simulink library "util_common_lib"  (R2014b)
settings: Solver=ode45  SolverMode=SingleTasking  StartTime=0.0  StopTime=10.0  RelTol=1e-3
undefined symbols (not defined in the file or in its folder): enum_boolean, sc_msgid, sc_start_rts_id, start
undefined symbols (not defined in the file): Initial_MET, slope, util_noise_generator_sample_time
libraries: simulink x13, util_info_lib x12, util_common_lib x5
settings Model: Creator=dviazzo  LastModifiedBy=mstewart

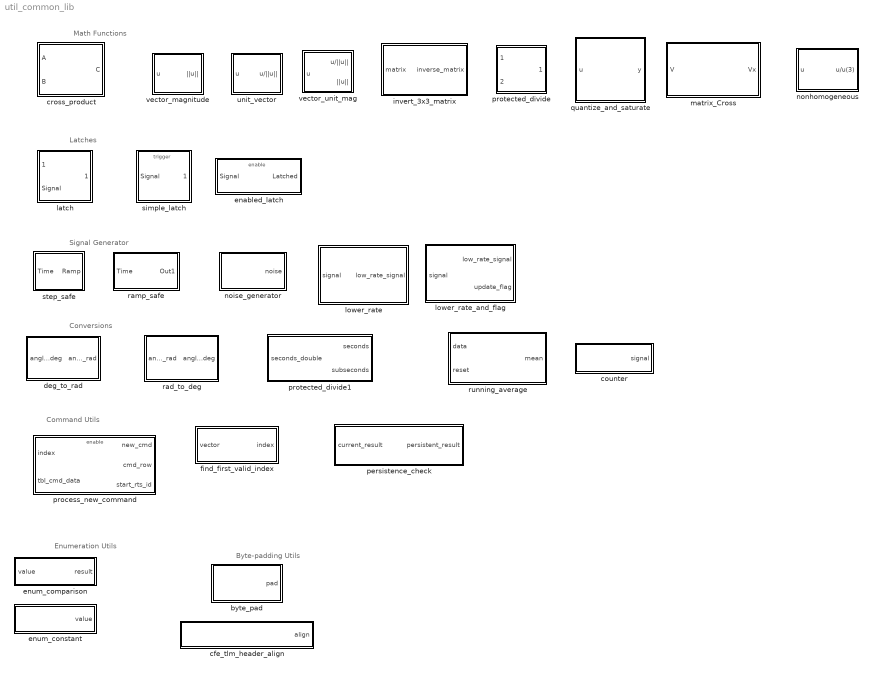
== system util_common_lib ==
  note: Enumeration Utils
  note: Command Utils
  note: Math Functions
  note: Latches
  note: Signal Generator
  note: Conversions
  note: Byte-padding Utils
  byte_pad : Subsystem  mask{n_bytes=1}
      mask prompts: n_bytes "Number of byes to pad"
      mask Display:
      | fprintf('pad %i bytes', n_bytes)
      | 
      | color('blue')
      | text(0.05,0.02,'moonex',...
      |  	'HorizontalAlignment','Left',...
      | 	'VerticalAlignment','bottom')
  cfe_tlm_header_align : Subsystem
      mask Display:
      | disp('cFE Telemetry Header Align');
      | 
      | color('blue')
      | text(0.05,0.02,'moonex',...
      |  	'HorizontalAlignment','Left',...
      | 	'VerticalAlignment','bottom')
  counter : Subsystem  TreatAsAtomicUnit=on  mask{n=0}
      mask prompts: n "Counter cycles (in ticks)"
      mask Display:
      | color('blue')
      | text(0.05,0.02,'MoonEx',...
      |  	'HorizontalAlignment','Left',...
      | 	'VerticalAlignment','bottom')
  cross_product : Subsystem
      mask Display:
      | text(.5,.5,'Cross\nProduct\nC = AxB', ...
      | 	'HorizontalAlignment','Center',...
      | 	'VerticalAlignment','middle')
      | color('blue')
      | text(0.05,0.02,'NASA',...
      |  	'HorizontalAlignment','Left',...
      | 	'VerticalAlignment','bottom')
  deg_to_rad : Subsystem
      mask Display:
      | disp('radians\ndegrees')
      | 
      | plot([.3 .7],[.47 .47])
      | 
      | color('blue')
      | text(0.05,0.02,'NASA',...
      |  	'HorizontalAlignment','Left',...
      | 	'VerticalAlignment','bottom')
  enabled_latch : Subsystem  mask{initial_output=0}
      mask prompts: initial_output "Initial Output Value"
      mask Display:
      | color('blue')
      | text(0.05,0.02,'NASA',...
      |  	'HorizontalAlignment','Left',...
      | 	'VerticalAlignment','bottom')
  enum_comparison : Subsystem  mask{comparison_type=~=, enum_type=enum_boolean, enum_value=FALSE}
      mask prompts: comparison_type "Relational Operator:"; enum_type "Enumeration Type:"; enum_value "Enumeration Value:"
      mask help:
      | Compares the incoming signal to an enumerated type.
      |
      | Once you change the enumeration type, the value selection will become disabled and you MUST close and reopen the dialog to reenable it.
      mask init:
      | rtw_data = get_param(gcb,'RTWData');  % Non-Persistent Data
      | user_data = get_param(gcb,'UserData'); % Persistent Data
      | 
      | mask_styles = get_param(gcb, 'MaskStyles');
      | 
      | if isempty(rtw_data)
      |     mask_styles{2} = user_data.type_popup;
      |     mask_styles{3} = user_data.value_popup;
      |     
      |     set_param(gcb, 'MaskStyles', mask_styles);
      |     set_param(gcb, 'enum_type', user_data.type);
      |     set_param(gcb, 'enum_value', user_data.value);
      |     
      |     if ~strcmp(gcb,'util_common_lib/enum_comparison')
      |         rtw_data.loaded = 'true';
      |     end
      |     set_param(gcb, 'RTWData', rtw_data);
      | else
      |     user_data.type_popup = mask_styles{2};
      |     user_data.value_popup = mask_styles{3};
      |     user_data.type = enum_type;
      |     user_data.value = enum_value;
      |     set_param(gcb, 'UserData', user_data);
      | end
      | 
      | mask_enables = get_param(gcb, 'MaskEnables');
      | 
      | % Make sure the user isn't selecting '...' on purpose.
      | if strcmp(enum_value, '...')
      |     if ~strcmp(mask_enables{3}, 'off')
      |         error('You must select a value.');
      |     end
      | else
      |     % Figure out the native type we're casting to
      |     enum_parents = superclasses(enum_type);
      |     bus_type = enum_parents{1};
      | 
      |     % Build up the constant string and update the inner compare block
      |     const_string = [ bus_type '(' enum_type '.' lower(enum_value) ')' ];
      |     set_param([gcb '/comparison'], 'const', const_string);
      |     set_param([gcb '/comparison'], 'relop', comparison_type);
      | end
      | 
      | clear rtw_data user_data mask_styles mask_enables enum_parents bus_type const_string
      mask TypeOptions comparison_type: == | ~=
      mask TypeOptions enum_type: enum_ap_state | enum_boolean | enum_burn_type | enum_mode | enum_reference_frame | enum_submode | enum_thruster_type
      mask Callback enum_type:
      | % Generate a list of enumeration files
      | nimbus_root = getenv('NIMBUS_ROOT');
      | enum_files = dir(fullfile(nimbus_root,'fsw','cmp','enums','*.m'));
      | % Extract the enum names into a cell array
      | enum_types = strrep({enum_files.name},'.m','');
      | 
      | user_data = get_param(gcb,'UserData');
      | 
      | % Build the popup of enum types
      | user_data.type_popup = ['popup(' strjoin(enum_types ,'|') ')'];
      | 
      | % Get current mask values
      | mask_values = get_param(gcb, 'MaskValues');
      | % Get a list of values the currently selected enumeration can take on
      | [~, enum_values] = enumeration(mask_values{2});
      | 
      | % Transpose enum_values and add in '...' so all enums share one field
      | enum_values = upper(['...' enum_values']);
      | % Construct the popup string for the enm values
      | user_data.value_popup = ['popup(' strjoin(enum_values, '|') ')'];
      | 
      | % Get the current mask styles and set the new enum type popup
      | mask_styles = get_param(gcb, 'MaskStyles');
      | mask_styles{2} = user_data.type_popup;
      | 
      | % If our determined values match the current style, the current popup
      | % is good and we can enable selection.
      | if strcmp(user_data.value_popup, mask_styles{3})
      |     set_param(gcb, 'MaskEnables', {'on';'on';'on'});
      | else
      |     % Otherwise disable the enum value popup and update its value. We have
      |     % to set the value to ... as an intermediate step to keep the window
      |     % from closing on us
      |     mask_styles{3} = user_data.value_popup;
      |     mask_values{3} = '...';
      |     set_param(gcb, 'MaskEnables', {'on';'on';'off'});
      |     set_param(gcb, 'MaskValues', mask_values);
      | end
      | 
      | % Send out the finalized mask styles
      | set_param(gcb, 'MaskStyles', mask_styles);
      | set_param(gcb, 'UserData', user_data);
      mask TypeOptions enum_value: ... | FALSE | TRUE
      mask Display: disp([comparison_type ' ' enum_value]);
  enum_constant : Subsystem  mask{enum_type=enum_boolean, enum_value=FALSE}
      mask prompts: enum_type "Enumeration Type:"; enum_value "Enumeration Value:"
      mask help:
      | Compares the incoming signal to an enumerated type.
      |
      | Once you change the enumeration type, the value selection will become disabled and you MUST close and reopen the dialog to reenable it.
      mask init:
      | rtw_data = get_param(gcb,'RTWData');  % Non-Persistent Data
      | user_data = get_param(gcb,'UserData'); % Persistent Data
      | 
      | mask_styles = get_param(gcb, 'MaskStyles');
      | 
      | if isempty(rtw_data)
      |     mask_styles{1} = user_data.type_popup;
      |     mask_styles{2} = user_data.value_popup;
      |     
      |     set_param(gcb, 'MaskStyles', mask_styles);
      |     set_param(gcb, 'enum_type', user_data.type);
      |     set_param(gcb, 'enum_value', user_data.value);
      |     
      |     if ~strcmp(gcb,'util_common_lib/enum_constant')
      |         rtw_data.loaded = 'true';
      |     end
      |     set_param(gcb, 'RTWData', rtw_data);
      | else
      |     user_data.type_popup = mask_styles{1};
      |     user_data.value_popup = mask_styles{2};
      |     user_data.type = enum_type;
      |     user_data.value = enum_value;
      |     set_param(gcb, 'UserData', user_data);
      | end
      | 
      | mask_enables = get_param(gcb, 'MaskEnables');
      | 
      | % Make sure the user isn't selecting '...' on purpose.
      | if strcmp(enum_value, '...')
      |     if ~strcmp(mask_enables{2}, 'off')
      |         error('You must select a value.');
      |     end
      | else
      |     % Figure out the native type we're casting to
      |     enum_parents = superclasses(enum_type);
      |     bus_type = enum_parents{1};
      | 
      |     % Build up the constant string and update the inner compare block
      |     const_string = [ bus_type '(' enum_type '.' lower(enum_value) ')' ];
      |     set_param([gcb '/constant'], 'Value', const_string);
      | end
      | 
      | 
      | clear rtw_data user_data mask_styles mask_enables enum_parents bus_type const_string
      mask TypeOptions enum_type: enum_ap_state | enum_boolean | enum_burn_type | enum_mode | enum_reference_frame | enum_submode | enum_thruster_type
      mask Callback enum_type:
      | % Generate a list of enumeration files
      | nimbus_root = getenv('NIMBUS_ROOT');
      | enum_files = dir(fullfile(nimbus_root,'fsw','cmp','enums','*.m'));
      | % Extract the enum names into a cell array
      | enum_types = strrep({enum_files.name},'.m','');
      | 
      | user_data = get_param(gcb,'UserData');
      | 
      | % Build the popup of enum types
      | user_data.type_popup = ['popup(' strjoin(enum_types ,'|') ')'];
      | 
      | % Get current mask values
      | mask_values = get_param(gcb, 'MaskValues');
      | % Get a list of values the currently selected enumeration can take on
      | [~, enum_values] = enumeration(mask_values{1});
      | 
      | % Transpose enum_values and add in '...' so all enums share one field
      | enum_values = upper(['...' enum_values']);
      | % Construct the popup string for the enm values
      | user_data.value_popup = ['popup(' strjoin(enum_values, '|') ')'];
      | 
      | % Get the current mask styles and set the new enum type popup
      | mask_styles = get_param(gcb, 'MaskStyles');
      | mask_styles{1} = user_data.type_popup;
      | 
      | % If our determined values match the current style, the current popup
      | % is good and we can enable selection.
      | if strcmp(user_data.value_popup, mask_styles{2})
      |     set_param(gcb, 'MaskEnables', {'on';'on'});
      | else
      |     % Otherwise disable the enum value popup and update its value. We have
      |     % to set the value to ... as an intermediate step to keep the window
      |     % from closing on us
      |     mask_styles{2} = user_data.value_popup;
      |     mask_values{2} = '...';
      |     set_param(gcb, 'MaskEnables', {'on';'off'});
      |     set_param(gcb, 'MaskValues', mask_values);
      | end
      | 
      | % Send out the finalized mask styles
      | set_param(gcb, 'MaskStyles', mask_styles);
      | set_param(gcb, 'UserData', user_data);
      mask TypeOptions enum_value: ... | FALSE | TRUE
      mask Display: disp(enum_value);
  find_first_valid_index : Subsystem  mask{vector_length=2}
      mask prompts: vector_length "Length of vector input"
      mask Display:
      | color('blue')
      | text(0.05,0.02,'MoonEx',...
      |  	'HorizontalAlignment','Left',...
      | 	'VerticalAlignment','bottom')
  invert_3x3_matrix : Subsystem
      mask Display:
      | disp('Inverse(A)\n(3x3)')
      | 
      | color('blue')
      | text(0.05,0.02,'NASA',...
      |  	'HorizontalAlignment','Left',...
      | 	'VerticalAlignment','bottom')
  latch : Subsystem  mask{Initial_Latch=[0 Initial_MET]}
      mask prompts: Initial_Latch "Initial Output Value"
      mask init:
      | if isempty(Initial_Latch)
      |    Initial_Latch = 0;
      | end
      mask Display:
      | color('blue')
      | text(0.05,0.02,'NASA',...
      |  	'HorizontalAlignment','Left',...
      | 	'VerticalAlignment','bottom')
  lower_rate : Subsystem  mask{counter_max=10, counter_init=0}
      mask prompts: counter_max "Counter maximum value (model freq / block freq)"; counter_init "Counter Initial Value"
      mask Display:
      | color('blue')
      | text(0.05,0.02,'MoonEx',...
      |  	'HorizontalAlignment','Left',...
      | 	'VerticalAlignment','bottom')
  lower_rate_and_flag : Subsystem  mask{counter_max=1, counter_init=[]}
      mask prompts: counter_max "Counter maximum value (model freq / block freq)"; counter_init "Counter initial value"
      mask Display:
      | color('blue')
      | text(0.05,0.02,'MoonEx',...
      |  	'HorizontalAlignment','Left',...
      | 	'VerticalAlignment','bottom')
  matrix_Cross : Subsystem
      mask Display:
      | text(.5,.5,'Cross\nMatrix\nV -> Vx', ...
      | 	'HorizontalAlignment','Center',...
      | 	'VerticalAlignment','middle')
      | color('blue')
      | text(0.05,0.02,'NASA',...
      |  	'HorizontalAlignment','Left',...
      | 	'VerticalAlignment','bottom')
  noise_generator : Subsystem  mask(noise_generator){std_dev=, bias=, seed=, on=1, sample_time=util_noise_generator_sample_time}
      mask prompts: std_dev "std deviation"; sample_time "sample time"
      mask help: Outputs a noise signal.
      mask init:
      | null_vector=zeros(size(std_dev));
      mask Display:
      | color('blue')
      | text(0.05,0.02,'NASA',...
      |  	'HorizontalAlignment','Left',...
      | 	'VerticalAlignment','bottom')
  nonhomogeneous : Subsystem
      mask Display:
      | color('blue')
      | text(0.05,0.02,'NASA',...
      |  	'HorizontalAlignment','Left',...
      | 	'VerticalAlignment','bottom')
  persistence_check : Subsystem  mask{persistence_limit=10}
      mask prompts: persistence_limit "Persistence Limit (counter initialize at zero)"
      mask Display:
      | color('blue')
      | text(0.05,0.02,'MoonEx',...
      |  	'HorizontalAlignment','Left',...
      | 	'VerticalAlignment','bottom')
  process_new_command : Subsystem  TreatAsAtomicUnit=on
      mask Display:
      | color('blue')
      | text(0.05,0.02,'MoonEx',...
      |  	'HorizontalAlignment','Left',...
      | 	'VerticalAlignment','bottom')
  protected_divide : Subsystem  mask{fault_value=0, tolerance=eps}
      mask prompts: fault_value "Fault value to be output when div by zero occurs"; tolerance "Tolerance for divisor below which fault is declared"
      mask Display:
      | color('blue')
      | text(0.05,0.02,'MoonEx',...
      |  	'HorizontalAlignment','Left',...
      | 	'VerticalAlignment','bottom')
      | 
      | color('black')
      | port_label('input', 1, '*')
      | port_label('input', 2, '/')
      | 
      | port_label('output', 1, '>')
      | 
      | disp('divide')
  protected_divide1 : Subsystem
      mask Display:
      | color('blue')
      | text(0.05,0.02,'MoonEx',...
      |  	'HorizontalAlignment','Left',...
      | 	'VerticalAlignment','bottom')
      | 
      | color('black')
      | port_label('input', 1, 't')
      | 
      | port_label('output', 1, 'secs')
      | port_label('output', 2, 'subs')
      | 
      | disp('6byte time')
  quantize_and_saturate : Subsystem  mask(PWL-Palette){RES=1, OPER=truncate, out_min=-inf, out_max=inf}
      mask prompts: RES "Resolution:"; OPER "Type"; out_min "Output Minimum"; out_max "Output Maximum"
      mask init:
      | x=[-5:.1:5];operator={'round';'fix';'floor';'ceil'};
      | y=feval(operator{OPER},x);
      | if(isfinite(out_max))
      |    y(find(y>3))=3;
      | end
      | if(isfinite(out_min))
      |    y(find(y<-3))=-3;
      | end
      | [xx,yy]=stairs(x,y);
      | set_param([gcb '/Type'],'Operator',operator{OPER});
      mask TypeOptions OPER: round | truncate | floor | ceil
      mask Display:
      | plot([0 0],[-4,4],[-4,4],[0 0],xx,yy)
      | color('blue')
      | text(1.5,-5,'NASA',...
      |  	'HorizontalAlignment','Left',...
      | 	'VerticalAlignment','bottom')
  rad_to_deg : Subsystem
      mask Display:
      | disp('degrees\nradians')
      | 
      | plot([.3 .7],[.47 .47])
      | 
      | color('blue')
      | text(0.05,0.02,'NASA',...
      |  	'HorizontalAlignment','Left',...
      | 	'VerticalAlignment','bottom')
  ramp_safe : Subsystem  mask(Ramp){slope=, start=, X0=, VectorParams1D=on}
      mask prompts: start "Start time:"; X0 "Initial output:"; VectorParams1D "Interpret vector parameters as 1-D"
      mask help: Output a ramp signal starting at the specified time.
      mask Display:
      | plot([0:10],[.001,.001,.001,.001,.001,1:6])
      | 
      | color('blue')
      | text(0.05,0.02,'NASA',...
      |  	'HorizontalAlignment','Left',...
      | 	'VerticalAlignment','bottom')
  running_average : Subsystem  mask{initial_mean=[0 0 0]}
      mask prompts: initial_mean "initial mean value:"
      mask Display:
      | color('blue')
      | text(0.05,0.02,'MoonEx',...
      |  	'HorizontalAlignment','Left',...
      | 	'VerticalAlignment','bottom')
  simple_latch : Subsystem
      mask Display:
      | color('blue')
      | text(0.05,0.02,'NASA',...
      |  	'HorizontalAlignment','Left',...
      | 	'VerticalAlignment','bottom')
  step_safe : Subsystem  mask{step_time=start, initial_value=0, final_value=slope}
      mask prompts: step_time "Step time:"; initial_value "Initial value:"; final_value "Final value:"
      mask Display:
      | plot([0,.5,.5,1],[.001,.001,.999,.999])
      | 
      | color('blue')
      | text(0.05,0.02,'NASA',...
      |  	'HorizontalAlignment','Left',...
      | 	'VerticalAlignment','bottom')
  unit_vector : Subsystem
      mask Display:
      | color('blue')
      | text(0.05,0.02,'NASA',...
      |  	'HorizontalAlignment','Left',...
      | 	'VerticalAlignment','bottom')
  vector_magnitude : Subsystem
      mask Display:
      | port_label('input',1,'u')
      | port_label('output',1,'||u||')
      | color('blue')
      | text(0.05,0.02,'NASA',...
      |  	'HorizontalAlignment','Left',...
      | 	'VerticalAlignment','bottom')
  vector_unit_mag : Subsystem
      mask Display:
      | color('blue')
      | text(0.05,0.02,'NASA',...
      |  	'HorizontalAlignment','Left',...
      | 	'VerticalAlignment','bottom')

== system util_common_lib/byte_pad ==
  note: Extremely explicit signal typing for uint8s of variable size for message padding
  Constant : Constant  Value=zeros(1,n_bytes)  OutDataTypeStr=uint8
  Data Type Conversion : DataTypeConversion  OutDataTypeStr=uint8
  Library Information : util_info_lib/Library Information  owner='NONE'
  pad : Outport
  wires:
  Constant/1 -> Data Type Conversion/1
  Data Type Conversion/1 -> pad/1

== system util_common_lib/cfe_tlm_header_align ==
  Constant : Constant  Value=zeros(1,4)  OutDataTypeStr=uint8
  Data Type Conversion : DataTypeConversion  OutDataTypeStr=uint8
  Library Information : util_info_lib/Library Information  owner='NONE'
  align : Outport
  wires:
  Data Type Conversion/1 -> align/1
  Constant/1 -> Data Type Conversion/1

== system util_common_lib/counter ==
  Bias : Bias  Bias=1
  Compare To Constant : simulink/Logic and Bit Operations/Compare To Constant  relop=>=  const=n  OutDataTypeStr=uint8
  Library Information : util_info_lib/Library Information  owner='NONE'
  Memory : Memory  X0=n  InheritSampleTime=on
  Switch6 : Switch  Criteria=u2 ~= 0  InputSameDT=on
  constant1 : Constant  Value=0
  signal : Outport
  wires:
  constant1/1 -> Switch6/1
  Bias/1 -> Compare To Constant/1, Switch6/3
  Compare To Constant/1 -> Switch6/2, signal/1
  Switch6/1 -> Memory/1
  Memory/1 -> Bias/1

== system util_common_lib/cross_product ==
  A : Inport
  B : Inport  Port=2
  Vector Concatenate : Concatenate  NumInputs=3
  Vector Concatenate1 : Concatenate
  i axis : Fcn  Expr=u(2)*u(6)-u(5)*u(3)
  j axis : Fcn  Expr=u(4)*u(3)-u(1)*u(6)
  k axis : Fcn  Expr=u(1)*u(5)-u(4)*u(2)
  C : Outport
  wires:
  B/1 -> Vector Concatenate1/2
  Vector Concatenate/1 -> C/1
  A/1 -> Vector Concatenate1/1
  k axis/1 -> Vector Concatenate/3
  j axis/1 -> Vector Concatenate/2
  i axis/1 -> Vector Concatenate/1
  Vector Concatenate1/1 -> k axis/1, j axis/1, i axis/1

== system util_common_lib/deg_to_rad ==
  angle_in_deg : Inport
  Gain : Gain  Gain=0.017453292519943295474371680598
  angle_in_rad : Outport
  wires:
  angle_in_deg/1 -> Gain/1
  Gain/1 -> angle_in_rad/1

== system util_common_lib/enabled_latch ==
  Signal : Inport
  Enable : EnablePort
  Latched : Outport  InitialOutput=initial_output
  wires:
  Signal/1 -> Latched/1

== system util_common_lib/enum_comparison ==
  value : Inport
  Library Information : util_info_lib/Library Information  owner='NONE'
  comparison : simulink/Logic and Bit Operations/Compare To Constant  relop=~=  const=uint8(enum_boolean.false)  OutDataTypeStr=boolean
  result : Outport
  wires:
  value/1 -> comparison/1
  comparison/1 -> result/1

== system util_common_lib/enum_constant ==
  Library Information : util_info_lib/Library Information  owner='NONE'
  constant : Constant  Value=uint8(enum_boolean.false)
  value : Outport
  wires:
  constant/1 -> value/1

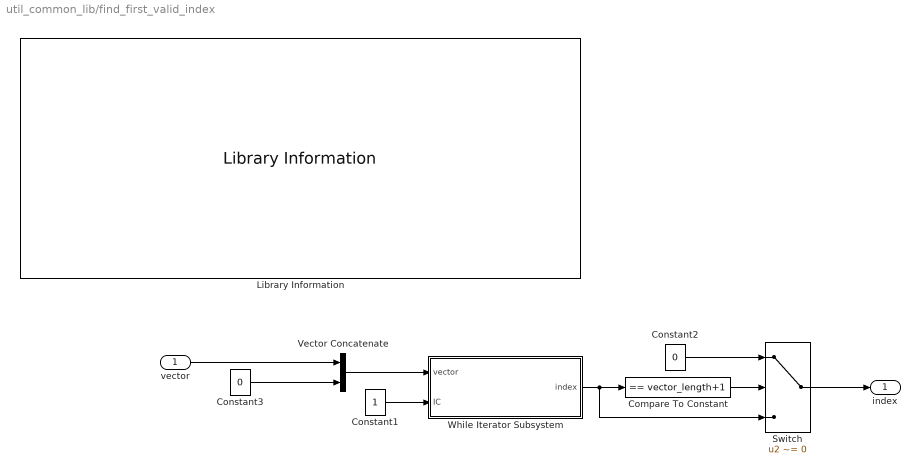
== system util_common_lib/find_first_valid_index ==
  vector : Inport
  Compare To Constant : simulink/Logic and Bit Operations/Compare To Constant  relop===  const=vector_length+1  OutDataTypeStr=boolean
  Constant1 : Constant  OutDataTypeStr=uint8
  Constant2 : Constant  Value=0  OutDataTypeStr=uint32
  Constant3 : Constant  Value=0  OutDataTypeStr=Inherit: Inherit via back propagation
  Library Information : util_info_lib/Library Information  owner='NONE'
  Switch : Switch  Criteria=u2 ~= 0
  Vector Concatenate : Concatenate
  While Iterator Subsystem : Subsystem  TreatAsAtomicUnit=on
  index : Outport
  wires:
  Constant3/1 -> Vector Concatenate/2
  Vector Concatenate/1 -> While Iterator Subsystem/1(vector)
  vector/1 -> Vector Concatenate/1
  Switch/1 -> index/1
  Constant2/1 -> Switch/1
  Compare To Constant/1 -> Switch/2
  While Iterator Subsystem/1(index) -> Compare To Constant/1, Switch/3
  Constant1/1 -> While Iterator Subsystem/2(IC)

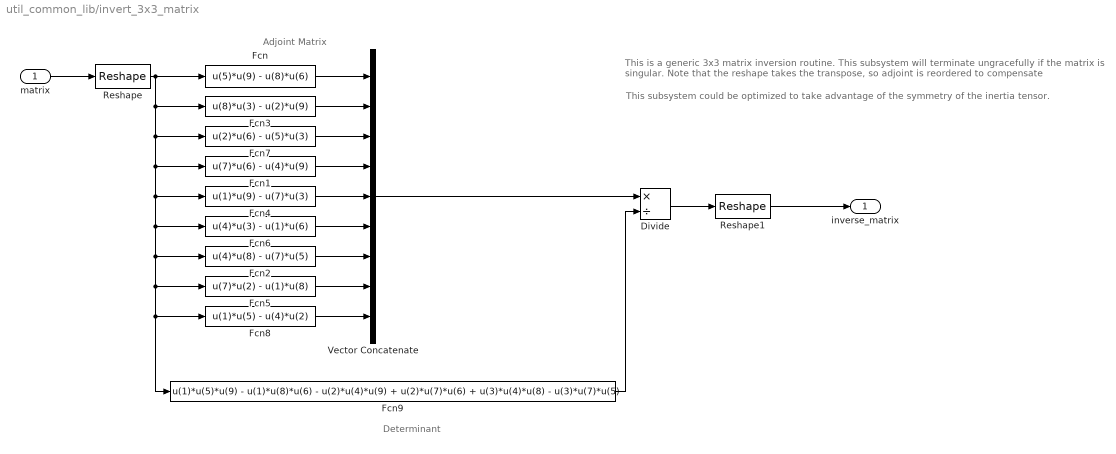
== system util_common_lib/invert_3x3_matrix ==
  note: Adjoint Matrix
  note: Determinant
  note: This is a generic 3x3 matrix inversion routine.
      | This subsystem will terminate ungracefully if the matrix is singular.
      | Note that the reshape takes the transpose, so adjoint is reordered to compensate
  note: This subsystem could be optimized to take advantage of the symmetry of the inertia tensor.
  matrix : Inport
  Divide : Product  Inputs=*/
  Fcn : Fcn  Expr=u(5)*u(9) - u(8)*u(6)
  Fcn1 : Fcn  Expr=u(7)*u(6) - u(4)*u(9)
  Fcn2 : Fcn  Expr=u(4)*u(8) - u(7)*u(5)
  Fcn3 : Fcn  Expr=u(8)*u(3) - u(2)*u(9)
  Fcn4 : Fcn  Expr=u(1)*u(9) - u(7)*u(3)
  Fcn5 : Fcn  Expr=u(7)*u(2) - u(1)*u(8)
  Fcn6 : Fcn  Expr=u(4)*u(3) - u(1)*u(6)
  Fcn7 : Fcn  Expr=u(2)*u(6) - u(5)*u(3)
  Fcn8 : Fcn  Expr=u(1)*u(5) - u(4)*u(2)
  Fcn9 : Fcn  Expr=u(1)*u(5)*u(9) - u(1)*u(8)*u(6) - u(2)*u(4)*u(9) + u(2)*u(7)*u(6) + u(3)*u(4)*u(8) - u(3)*u(7)*u(5)
  Reshape : Reshape  OutputDimensionality=Row vector (2-D)
  Reshape1 : Reshape  OutputDimensionality=Customize  OutputDimensions=[3,3]
  Vector Concatenate : Concatenate  NumInputs=9
  inverse_matrix : Outport
  wires:
  matrix/1 -> Reshape/1
  Fcn9/1 -> Divide/2
  Reshape/1 -> Fcn/1, Fcn3/1, Fcn7/1, Fcn1/1, Fcn4/1, Fcn6/1, Fcn2/1, Fcn5/1, Fcn9/1, Fcn8/1
  Divide/1 -> Reshape1/1
  Reshape1/1 -> inverse_matrix/1
  Fcn/1 -> Vector Concatenate/1
  Fcn3/1 -> Vector Concatenate/2
  Fcn7/1 -> Vector Concatenate/3
  Fcn1/1 -> Vector Concatenate/4
  Fcn4/1 -> Vector Concatenate/5
  Fcn6/1 -> Vector Concatenate/6
  Fcn2/1 -> Vector Concatenate/7
  Fcn5/1 -> Vector Concatenate/8
  Fcn8/1 -> Vector Concatenate/9
  Vector Concatenate/1 -> Divide/1

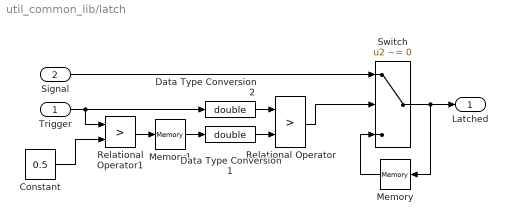
== system util_common_lib/latch ==
  Trigger : Inport
  Signal : Inport  Port=2
  Constant : Constant  Value=0.5
  Data Type Conversion1 : DataTypeConversion  OutDataTypeStr=double
  Data Type Conversion2 : DataTypeConversion  OutDataTypeStr=double
  Memory : Memory  X0=Initial_Latch  InheritSampleTime=on
  Memory1 : Memory  InheritSampleTime=on
  Relational Operator : RelationalOperator  Operator=>  OutDataTypeStr=boolean
  Relational Operator1 : RelationalOperator  Operator=>  OutDataTypeStr=boolean
  Switch : Switch  Criteria=u2 ~= 0  InputSameDT=on
  Latched : Outport
  wires:
  Trigger/1 -> Data Type Conversion2/1, Relational Operator1/1
  Relational Operator1/1 -> Memory1/1
  Memory/1 -> Switch/3
  Signal/1 -> Switch/1
  Switch/1 -> Latched/1, Memory/1
  Constant/1 -> Relational Operator1/2
  Data Type Conversion2/1 -> Relational Operator/1
  Memory1/1 -> Data Type Conversion1/1
  Data Type Conversion1/1 -> Relational Operator/2
  Relational Operator/1 -> Switch/2

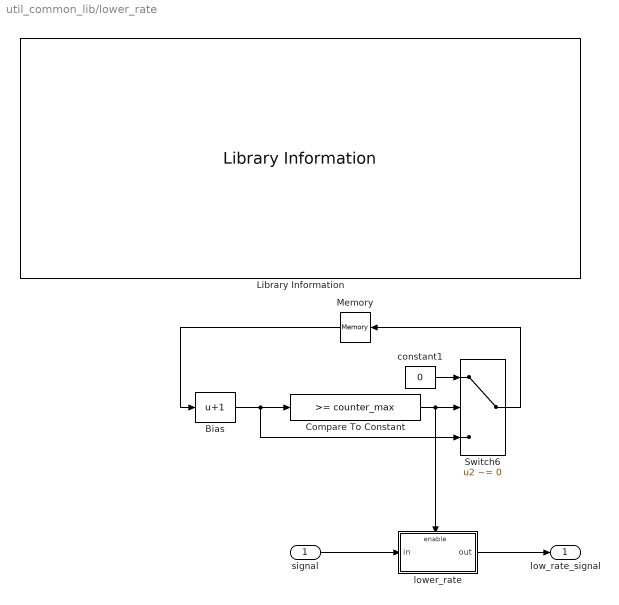
== system util_common_lib/lower_rate ==
  signal : Inport
  Bias : Bias  Bias=1
  Compare To Constant : simulink/Logic and Bit Operations/Compare To Constant  relop=>=  const=counter_max  OutDataTypeStr=uint8
  Library Information : util_info_lib/Library Information  owner='NONE'
  Memory : Memory  X0=counter_init  InheritSampleTime=on
  Switch6 : Switch  Criteria=u2 ~= 0  InputSameDT=on
  constant1 : Constant  Value=0
  lower_rate : Subsystem  TreatAsAtomicUnit=on
  low_rate_signal : Outport
  wires:
  Memory/1 -> Bias/1
  Switch6/1 -> Memory/1
  Compare To Constant/1 -> Switch6/2, lower_rate/Enable
  Bias/1 -> Switch6/3, Compare To Constant/1
  constant1/1 -> Switch6/1
  signal/1 -> lower_rate/1(in)
  lower_rate/1(out) -> low_rate_signal/1

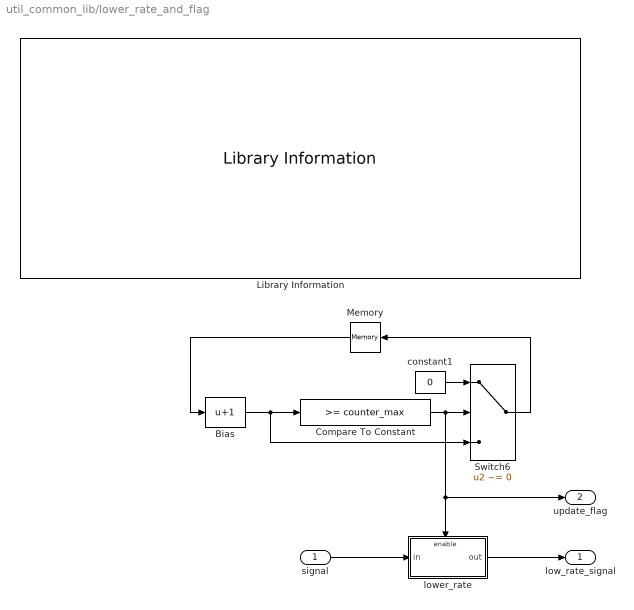
== system util_common_lib/lower_rate_and_flag ==
  signal : Inport
  Bias : Bias  Bias=1
  Compare To Constant : simulink/Logic and Bit Operations/Compare To Constant  relop=>=  const=counter_max  OutDataTypeStr=uint8
  Library Information : util_info_lib/Library Information  owner='NONE'
  Memory : Memory  X0=counter_init  InheritSampleTime=on
  Switch6 : Switch  Criteria=u2 ~= 0  InputSameDT=on
  constant1 : Constant  Value=0
  lower_rate : Subsystem  TreatAsAtomicUnit=on
  low_rate_signal : Outport
  update_flag : Outport  Port=2
  wires:
  Memory/1 -> Bias/1
  Switch6/1 -> Memory/1
  Compare To Constant/1 -> Switch6/2, update_flag/1, lower_rate/Enable
  Bias/1 -> Switch6/3, Compare To Constant/1
  constant1/1 -> Switch6/1
  signal/1 -> lower_rate/1(in)
  lower_rate/1(out) -> low_rate_signal/1

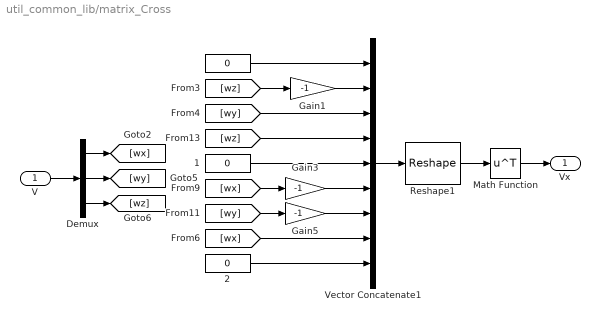
== system util_common_lib/matrix_Cross ==
  V : Inport
  "     " : Constant  Value=0
  "     1" : Constant  Value=0
  "     2" : Constant  Value=0
  Demux : Demux  Outputs=[1 1 1]
  Gain1 : Gain  Gain=-1
  Gain3 : Gain  Gain=-1
  Gain5 : Gain  Gain=-1
  Math Function : Math  Operator=transpose  SaturateOnIntegerOverflow=on
  Reshape1 : Reshape  OutputDimensionality=Customize  OutputDimensions=[3,3]
  Vector Concatenate1 : Concatenate  NumInputs=9
  Vx : Outport
  wires:
  "     "/1 -> Vector Concatenate1/1
  Gain1/1 -> Vector Concatenate1/2
  [wy] -> Vector Concatenate1/3
  [wz] -> Vector Concatenate1/4
  "     1"/1 -> Vector Concatenate1/5
  Gain3/1 -> Vector Concatenate1/6
  Gain5/1 -> Vector Concatenate1/7
  [wx] -> Vector Concatenate1/8
  "     2"/1 -> Vector Concatenate1/9
  [wz] -> Gain1/1
  Reshape1/1 -> Math Function/1
  Vector Concatenate1/1 -> Reshape1/1
  [wy] -> Gain5/1
  [wx] -> Gain3/1
  Demux/1 -> [wx]
  Demux/2 -> [wy]
  Demux/3 -> [wz]
  Math Function/1 -> Vx/1
  V/1 -> Demux/1

== system util_common_lib/noise_generator ==
  Constant : Constant  Value=null_vector
  Constant1 : Constant  Value=on
  Random Number : RandomNumber  Mean=bias  Variance=std_dev.^2  Seed=seed  SampleTime=sample_time
  Switch : Switch  Criteria=u2 > Threshold
  noise : Outport
  wires:
  Constant1/1 -> Switch/2
  Constant/1 -> Switch/3
  Random Number/1 -> Switch/1
  Switch/1 -> noise/1

== system util_common_lib/nonhomogeneous ==
  u : Inport
  If : If  IfExpression=u1 ~= 0
  Merge : Merge
  Selector : Selector  InputPortWidth=3  Indices=[3]
  Selector1 : Selector  InputPortWidth=3  Indices=[1 2]
  divide by zero detected : util_common_lib/vector_unit_mag/divide by zero detected
  normalize : util_common_lib/vector_unit_mag/If Action Subsystem
  u/u(3) : Outport
  wires:
  Merge/1 -> u/u(3)/1
  divide by zero detected/1 -> Merge/2
  normalize/1 -> Merge/1
  Selector/1 -> normalize/2, If/1
  If/1 -> normalize/Action
  If/2 -> divide by zero detected/Action
  u/1 -> Selector1/1, Selector/1
  Selector1/1 -> normalize/1, divide by zero detected/1

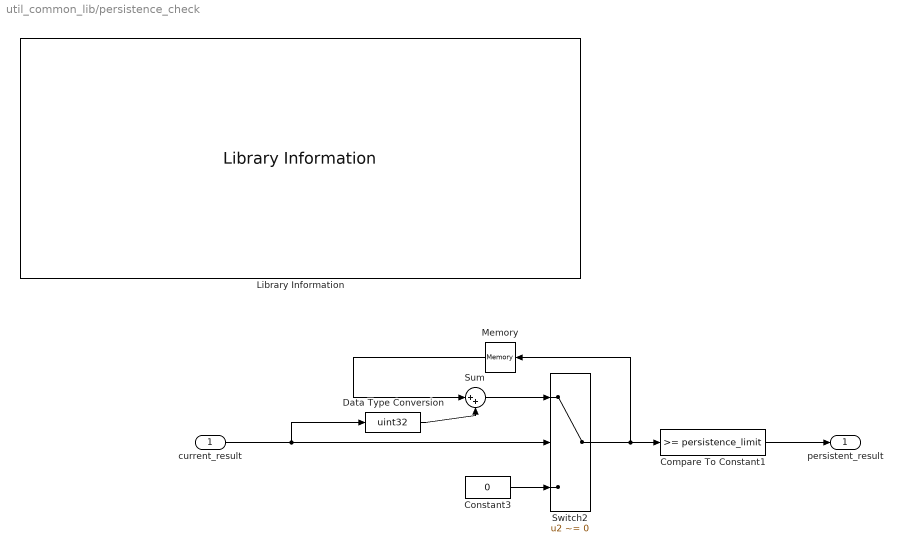
== system util_common_lib/persistence_check ==
  current_result : Inport
  Compare To Constant1 : simulink/Logic and Bit Operations/Compare To Constant  relop=>=  const=persistence_limit  OutDataTypeStr=boolean
  Constant3 : Constant  Value=0  OutDataTypeStr=uint32
  Data Type Conversion : DataTypeConversion  OutDataTypeStr=uint32
  Library Information : util_info_lib/Library Information  owner='NONE'
  Memory : Memory  InheritSampleTime=on
  Sum : Sum  Inputs=|++
  Switch2 : Switch  Criteria=u2 ~= 0  InputSameDT=on
  persistent_result : Outport
  wires:
  Compare To Constant1/1 -> persistent_result/1
  Constant3/1 -> Switch2/3
  Sum/1 -> Switch2/1
  Memory/1 -> Sum/1
  Switch2/1 -> Memory/1, Compare To Constant1/1
  Data Type Conversion/1 -> Sum/2
  current_result/1 -> Data Type Conversion/1, Switch2/2

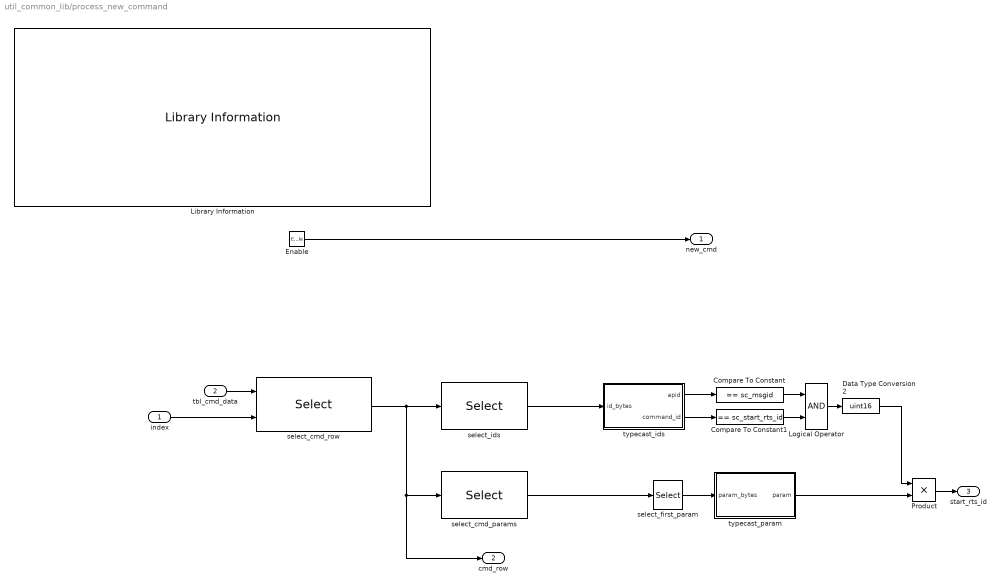
== system util_common_lib/process_new_command ==
  index : Inport
  tbl_cmd_data : Inport  Port=2
  Enable : EnablePort  ShowOutputPort=on
  Compare To Constant : simulink/Logic and Bit Operations/Compare To Constant  relop===  const=sc_msgid  OutDataTypeStr=boolean
  Compare To Constant1 : simulink/Logic and Bit Operations/Compare To Constant  relop===  const=sc_start_rts_id  OutDataTypeStr=boolean
  Data Type Conversion2 : DataTypeConversion  OutDataTypeStr=uint16
  Library Information : util_info_lib/Library Information  owner='NONE'
  Logical Operator : Logic  AllPortsSameDT=off  OutDataTypeStr=boolean
  Product : Product  OutDataTypeStr=uint16
  select_cmd_params : Selector  InputPortWidth=sc_tbl_cmd_size  Indices=sc_params_index
  select_cmd_row : Selector  NumberOfDimensions=2  InputPortWidth=3  IndexOptions=Index vector (port),Select all  Indices=[1 3],1  OutputSizes=1,1
  select_first_param : Selector  InputPortWidth=sc_params_size  Indices=[1 2]
  select_ids : Selector  InputPortWidth=sc_tbl_cmd_size  Indices=sc_ids_index
  typecast_ids : Subsystem
  typecast_param : Subsystem
  new_cmd : Outport  OutputWhenDisabled=reset  InitialOutput=0
  cmd_row : Outport  Port=2
  start_rts_id : Outport  Port=3  OutputWhenDisabled=reset  InitialOutput=0
  wires:
  select_ids/1 -> typecast_ids/1(id_bytes)
  typecast_ids/2(command_id) -> Compare To Constant1/1
  typecast_ids/1(apid) -> Compare To Constant/1
  select_cmd_row/1 -> select_cmd_params/1, cmd_row/1, select_ids/1
  tbl_cmd_data/1 -> select_cmd_row/1
  index/1 -> select_cmd_row/2
  Compare To Constant/1 -> Logical Operator/1
  Compare To Constant1/1 -> Logical Operator/2
  select_cmd_params/1 -> select_first_param/1
  select_first_param/1 -> typecast_param/1(param_bytes)
  Logical Operator/1 -> Data Type Conversion2/1
  typecast_param/1(param) -> Product/2
  Data Type Conversion2/1 -> Product/1
  Product/1 -> start_rts_id/1
  Enable/1 -> new_cmd/1

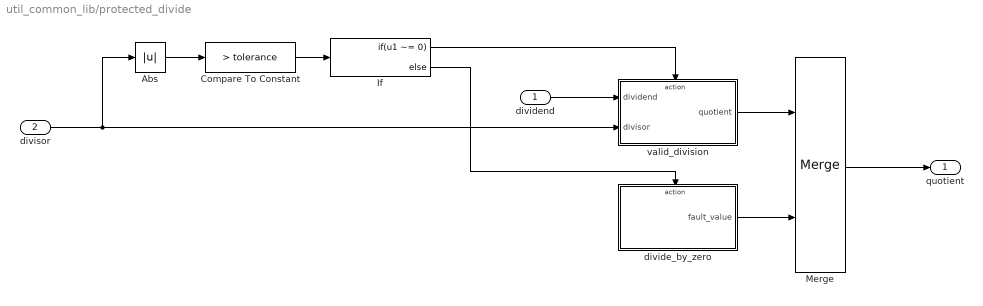
== system util_common_lib/protected_divide ==
  dividend : Inport
  divisor : Inport  Port=2
  Abs : Abs
  Compare To Constant : simulink/Logic and Bit Operations/Compare To Constant  relop=>  const=tolerance  OutDataTypeStr=boolean
  If : If  IfExpression=u1 ~= 0
  Merge : Merge
  divide_by_zero : Subsystem  TreatAsAtomicUnit=on
  valid_division : Subsystem  TreatAsAtomicUnit=on
  quotient : Outport
  wires:
  If/1 -> valid_division/Action
  valid_division/1(quotient) -> Merge/1
  divide_by_zero/1(fault_value) -> Merge/2
  If/2 -> divide_by_zero/Action
  divisor/1 -> Abs/1, valid_division/2(divisor)
  Compare To Constant/1 -> If/1
  dividend/1 -> valid_division/1(dividend)
  Merge/1 -> quotient/1
  Abs/1 -> Compare To Constant/1

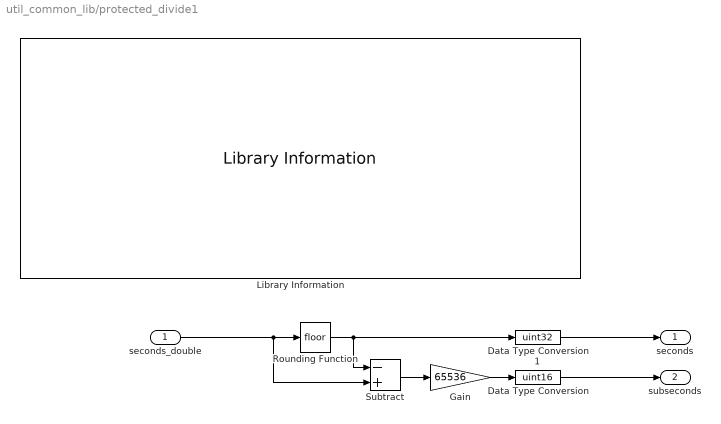
== system util_common_lib/protected_divide1 ==
  seconds_double : Inport
  Data Type Conversion : DataTypeConversion  OutDataTypeStr=uint16  RndMeth=Round
  Data Type Conversion1 : DataTypeConversion  OutDataTypeStr=uint32
  Gain : Gain  Gain=65536
  Library Information : util_info_lib/Library Information  owner='NONE'
  Rounding Function : Rounding
  Subtract : Sum  Inputs=-+
  seconds : Outport
  subseconds : Outport  Port=2
  wires:
  Gain/1 -> Data Type Conversion/1
  Rounding Function/1 -> Data Type Conversion1/1, Subtract/1
  Subtract/1 -> Gain/1
  seconds_double/1 -> Subtract/2, Rounding Function/1
  Data Type Conversion1/1 -> seconds/1
  Data Type Conversion/1 -> subseconds/1

== system util_common_lib/quantize_and_saturate ==
  u : Inport
  Resolution : Constant  Value=RES
  Saturation1 : Saturate  UpperLimit=out_max  LowerLimit=out_min
  Type : Rounding  Operator=fix
  div : Product  Inputs=*/  SaturateOnIntegerOverflow=on  RndMeth=Zero  InputSameDT=on  OutDataTypeStr=Inherit: Same as first input
  mul : Product  SaturateOnIntegerOverflow=on  RndMeth=Zero  InputSameDT=on  OutDataTypeStr=Inherit: Same as first input
  y : Outport
  wires:
  mul/1 -> Saturation1/1
  u/1 -> div/1
  Resolution/1 -> mul/2, div/2
  Type/1 -> mul/1
  div/1 -> Type/1
  Saturation1/1 -> y/1

== system util_common_lib/rad_to_deg ==
  angle_in_rad : Inport
  Gain : Gain  Gain=57.295779513082322864647721871734
  angle_in_deg : Outport
  wires:
  Gain/1 -> angle_in_deg/1
  angle_in_rad/1 -> Gain/1

== system util_common_lib/ramp_safe ==
  Time : Inport
  Constant : Constant  Value=start
  Constant1 : Constant  Value=X0
  Output : Sum  Inputs=|++  SaturateOnIntegerOverflow=on  InputSameDT=on  OutDataTypeStr=Inherit: Same as first input
  Product : Product  SaturateOnIntegerOverflow=on  InputSameDT=on  OutDataTypeStr=Inherit: Same as first input
  Sum : Sum  Inputs=|+-  SaturateOnIntegerOverflow=on  InputSameDT=on  OutDataTypeStr=Inherit: Same as first input
  step_safe : util_common_lib/step_safe  step_time=start  initial_value=0  final_value=slope
  Out1 : Outport
  wires:
  Time/1 -> Sum/1, step_safe/1
  Constant/1 -> Sum/2
  Sum/1 -> Product/2
  Output/1 -> Out1/1
  Constant1/1 -> Output/2
  Product/1 -> Output/1
  step_safe/1 -> Product/1

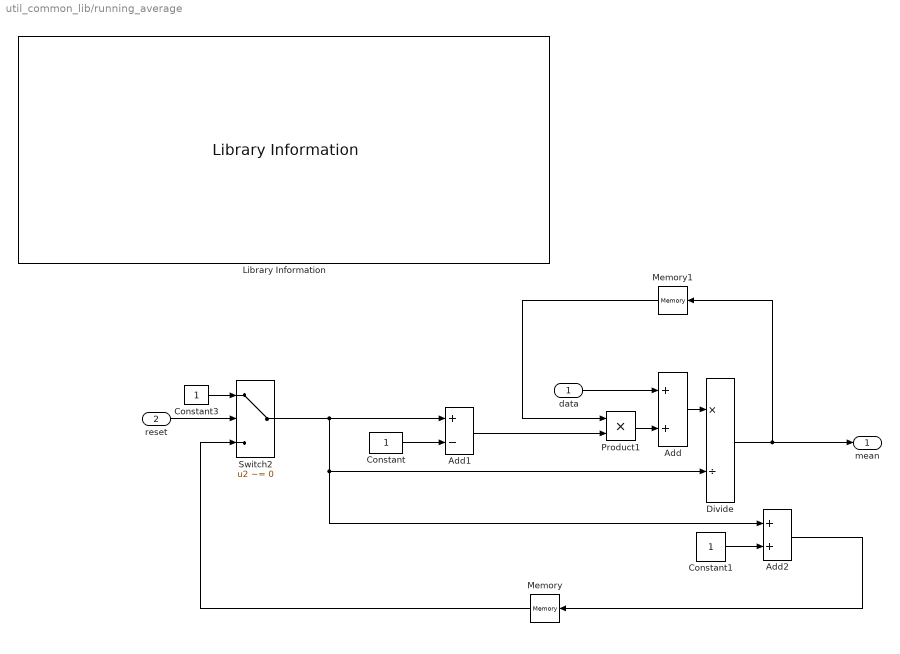
== system util_common_lib/running_average ==
  data : Inport
  reset : Inport  Port=2
  Add : Sum
  Add1 : Sum  Inputs=+-
  Add2 : Sum
  Constant : Constant
  Constant1 : Constant
  Constant3 : Constant
  Divide : Product  Inputs=*/
  Library Information : util_info_lib/Library Information  owner='NONE'
  Memory : Memory  X0=1  InheritSampleTime=on
  Memory1 : Memory  X0=initial_mean  InheritSampleTime=on
  Product1 : Product  RndMeth=Zero
  Switch2 : Switch  Criteria=u2 ~= 0  Threshold=1
  mean : Outport
  wires:
  Divide/1 -> mean/1, Memory1/1
  Constant1/1 -> Add2/2
  Add2/1 -> Memory/1
  Constant/1 -> Add1/2
  data/1 -> Add/1
  Add1/1 -> Product1/2
  Memory1/1 -> Product1/1
  Product1/1 -> Add/2
  Add/1 -> Divide/1
  reset/1 -> Switch2/2
  Constant3/1 -> Switch2/1
  Switch2/1 -> Add1/1, Divide/2, Add2/1
  Memory/1 -> Switch2/3

== system util_common_lib/simple_latch ==
  Signal : Inport
  Trigger : TriggerPort
  Latched : Outport
  wires:
  Signal/1 -> Latched/1

== system util_common_lib/step_safe ==
  Time : Inport
  Constant : Constant  Value=step_time
  Constant1 : Constant  Value=initial_value
  Constant2 : Constant  Value=final_value
  Relational Operator : RelationalOperator  Operator=<  OutDataTypeStr=boolean
  Switch : Switch  Criteria=u2 > Threshold  Threshold=0.5
  Ramp : Outport
  wires:
  Switch/1 -> Ramp/1
  Time/1 -> Relational Operator/1
  Constant2/1 -> Switch/3
  Constant1/1 -> Switch/1
  Relational Operator/1 -> Switch/2
  Constant/1 -> Relational Operator/2

== system util_common_lib/unit_vector ==
  u : Inport
  Terminator : Terminator
  vector_unit_mag : util_common_lib/vector_unit_mag  SystemSampleTime=-1
  u/||u|| : Outport
  wires:
  vector_unit_mag/2 -> Terminator/1
  vector_unit_mag/1 -> u/||u||/1
  u/1 -> vector_unit_mag/1

== system util_common_lib/vector_magnitude ==
  u : Inport
  Dot Product : DotProduct  InputSameDT=on  OutDataTypeStr=Inherit: Inherit via internal rule
  Math Function : Math  Operator=sqrt  SaturateOnIntegerOverflow=on
  ||u|| : Outport
  wires:
  Math Function/1 -> ||u||/1
  Dot Product/1 -> Math Function/1
  u/1 -> Dot Product/1, Dot Product/2

== system util_common_lib/vector_unit_mag ==
  u : Inport
  If : If  IfExpression=u1 ~= 0
  If Action Subsystem : Subsystem  TreatAsAtomicUnit=on
  Merge : Merge
  divide by zero detected : Subsystem  TreatAsAtomicUnit=on
  vector_magnitude : util_common_lib/vector_magnitude  SystemSampleTime=-1
  u/||u|| : Outport
  ||u|| : Outport  Port=2
  wires:
  Merge/1 -> u/||u||/1
  divide by zero detected/1(Out1) -> Merge/2
  If Action Subsystem/1(Out1) -> Merge/1
  If/2 -> divide by zero detected/Action
  If/1 -> If Action Subsystem/Action
  vector_magnitude/1 -> ||u||/1, If Action Subsystem/2(In2), If/1
  u/1 -> vector_magnitude/1, divide by zero detected/1(In1), If Action Subsystem/1(In1)

== system util_common_lib/find_first_valid_index/While Iterator Subsystem ==
  vector : Inport
  IC : Inport  Port=2
  Compare To Zero : simulink/Logic and Bit Operations/Compare To Zero  relop===  OutDataTypeStr=boolean
  Selector : Selector  IndexOptions=Index vector (port)  Indices=[1 3]
  While Iterator : WhileIterator  MaxIters=vector_length+1  ShowIterationPort=on
  index : Outport
  wires:
  While Iterator/1 -> index/1, Selector/2
  vector/1 -> Selector/1
  Selector/1 -> Compare To Zero/1
  Compare To Zero/1 -> While Iterator/1
  IC/1 -> While Iterator/2

== system util_common_lib/lower_rate/lower_rate ==
  in : Inport
  Enable : EnablePort
  out : Outport
  wires:
  in/1 -> out/1

== system util_common_lib/lower_rate_and_flag/lower_rate ==
  in : Inport
  Enable : EnablePort
  out : Outport
  wires:
  in/1 -> out/1

== system util_common_lib/process_new_command/typecast_ids ==
  id_bytes : Inport
  Bitwise Operator : simulink/Logic and Bit Operations/Bitwise Operator  logicop=OR  UseBitMask=off  NumInputPorts=2  BitMask=bin2dec('11011001')  BitMaskRealWorld=Stored Integer
  Bitwise Operator1 : simulink/Logic and Bit Operations/Bitwise Operator  logicop=OR  UseBitMask=off  NumInputPorts=2  BitMask=bin2dec('11011001')  BitMaskRealWorld=Stored Integer
  Data Type Conversion : DataTypeConversion  OutDataTypeStr=uint16
  Demux : Demux
  Shift Arithmetic : ArithShift  BitShiftNumber=8  BitShiftDirection=Left
  Shift Arithmetic1 : ArithShift  BitShiftNumber=8  BitShiftDirection=Left
  apid : Outport
  command_id : Outport  Port=2
  wires:
  id_bytes/1 -> Data Type Conversion/1
  Data Type Conversion/1 -> Demux/1
  Demux/2 -> Shift Arithmetic/1
  Demux/4 -> Shift Arithmetic1/1
  Shift Arithmetic1/1 -> Bitwise Operator/2
  Demux/3 -> Bitwise Operator/1
  Shift Arithmetic/1 -> Bitwise Operator1/2
  Demux/1 -> Bitwise Operator1/1
  Bitwise Operator/1 -> command_id/1
  Bitwise Operator1/1 -> apid/1

== system util_common_lib/process_new_command/typecast_param ==
  param_bytes : Inport
  Bitwise Operator1 : simulink/Logic and Bit Operations/Bitwise Operator  logicop=OR  UseBitMask=off  NumInputPorts=2  BitMask=bin2dec('11011001')  BitMaskRealWorld=Stored Integer
  Data Type Conversion : DataTypeConversion  OutDataTypeStr=uint16
  Demux : Demux  Outputs=2
  Shift Arithmetic : ArithShift  BitShiftNumber=8  BitShiftDirection=Left
  param : Outport
  wires:
  Bitwise Operator1/1 -> param/1
  Demux/1 -> Bitwise Operator1/1
  Shift Arithmetic/1 -> Bitwise Operator1/2
  Demux/2 -> Shift Arithmetic/1
  Data Type Conversion/1 -> Demux/1
  param_bytes/1 -> Data Type Conversion/1

== system util_common_lib/protected_divide/divide_by_zero ==
  Action Port : ActionPort  ActionType=else
  Constant6 : Constant  Value=fault_value
  fault_value : Outport  InitialOutput=fault_value
  wires:
  Constant6/1 -> fault_value/1

== system util_common_lib/protected_divide/valid_division ==
  dividend : Inport
  divisor : Inport  Port=2
  Action Port : ActionPort  ActionType=then
  Divide1 : Product  Inputs=*/
  quotient : Outport
  wires:
  dividend/1 -> Divide1/1
  divisor/1 -> Divide1/2
  Divide1/1 -> quotient/1

== system util_common_lib/vector_unit_mag/If Action Subsystem ==
  In1 : Inport
  In2 : Inport  Port=2
  Action Port : ActionPort
  Divide : Product  Inputs=*/  InputSameDT=on
  Out1 : Outport
  wires:
  Divide/1 -> Out1/1
  In2/1 -> Divide/2
  In1/1 -> Divide/1

== system util_common_lib/vector_unit_mag/divide by zero detected ==
  In1 : Inport
  Action Port : ActionPort
  Out1 : Outport
  wires:
  In1/1 -> Out1/1
